simulink model "MIL4L3_SW6_V1_20220211"  (R2018b)
settings: Solver=FixedStepAuto  StartTime=0.0  StopTime=inf  FixedStep=0.001  RelTol=1e-3
PreLoadFcn:
  | A0_MILtest;
undefined symbols (not defined in the file or in its folder): Clb_ICADirect_LaneDisp_StateFive, Clb_ICADirect_LaneDisp_StateFour, Clb_ICADirect_LaneDisp_StateOne, Clb_ICADirect_LaneDisp_StateThree, Clb_ICADirect_LaneDisp_StateTwo, Clb_ICADirect_LaneDisp_StateZero, Clb_ICADirect_LaneDispSW, Clb_ICADirect_TrnLghtsCom_Switch, Clb_ICADirect_TrnLghtsCom_Value, Clb_ICADirect_TrnLghtsCrtl_Inhb, IMAP_Clb_ACU_Driver_Belt, IMAP_Clb_ACU_Driver_Belt_Over, IMAP_Clb_ACU_Passenger_Belt, IMAP_Clb_ACU_Passenger_Belt_Over, IMAP_Clb_ACU_RearLeft_Belt, IMAP_Clb_ACU_RearLeft_Belt_Over, IMAP_Clb_ACU_RearMiddle_Belt, IMAP_Clb_ACU_RearMiddle_Belt_Over, IMAP_Clb_ACU_RearRight_Belt, IMAP_Clb_ACU_RearRight_Belt_Over, IMAP_Clb_AEB_Switch, IMAP_Clb_AEB_Switch_Over, IMAP_Clb_ALC_TLC_Mode, IMAP_Clb_ALC_TLC_Mode_Over, IMAP_Clb_BCM_Battery_Voltage, IMAP_Clb_BCM_Battery_Voltage_Over, IMAP_Clb_BCM_BrakeLamp_State, IMAP_Clb_BCM_BrakeLamp_State_Over, IMAP_Clb_BCM_CHMSL_Status, IMAP_Clb_BCM_CHMSL_Status_Over, IMAP_Clb_BCM_Door_Lock_State, IMAP_Clb_BCM_Door_Lock_State_Over, IMAP_Clb_BCM_FrontWiper_State, IMAP_Clb_BCM_FrontWiper_State_Over, IMAP_Clb_BCM_FrontWiper_Switch, IMAP_Clb_BCM_FrontWiper_Switch_Over, IMAP_Clb_BCM_HazardLamp, IMAP_Clb_BCM_HazardLamp_Over, IMAP_Clb_BCM_HazardLamp_Switch, IMAP_Clb_BCM_HazardLamp_Switch_Over, IMAP_Clb_BCM_HighBeam_State, IMAP_Clb_BCM_HighBeam_State_Over, IMAP_Clb_BCM_Ignition_State, IMAP_Clb_BCM_Ignition_State_Over, IMAP_Clb_BCM_IHBC_Enabled, IMAP_Clb_BCM_IHBC_Enabled_Over, IMAP_Clb_BCM_Left_Light, IMAP_Clb_BCM_Left_Light_Over, IMAP_Clb_BCM_LeftTurn_Switch, IMAP_Clb_BCM_LeftTurn_Switch_Over, IMAP_Clb_BCM_LF_Door_State, IMAP_Clb_BCM_LF_Door_State_Over, IMAP_Clb_BCM_LowBeam_State, IMAP_Clb_BCM_LowBeam_State_Over, IMAP_Clb_BCM_LR_Door_State, IMAP_Clb_BCM_LR_Door_State_Over, IMAP_Clb_BCM_RF_Door_State, IMAP_Clb_BCM_RF_Door_State_Over, IMAP_Clb_BCM_Right_Light, IMAP_Clb_BCM_Right_Light_Over ... (+547)
libraries: CarMaker4SL x2153, simulink x292, dspstat3 x3, canmsglib x2, simulink_extras x1
(part 17 of 52)

== system MIL4L3_SW6_V1_20220211/CarMaker/VehicleControl/SDFADataLog/Subsystem53 ==
  BusCreator : BusCreator  Inputs=10
  Data Type Conversion{1..3,92} (4 alike) : DataTypeConversion  OutDataTypeStr=single
  Ground{,1..5} (6 alike) : Ground
  Read CM Dict1 : CarMaker4SL/Read CM Dict  xname=User.IO.Out.Width_S2_002  xsync=off
  Read CM Dict2 : CarMaker4SL/Read CM Dict  xname=User.IO.Out.Width_S2_003  xsync=off
  Read CM Dict3 : CarMaker4SL/Read CM Dict  xname=User.IO.Out.Width_S2_004  xsync=off
  Read CM Dict5 : CarMaker4SL/Read CM Dict  xname=User.IO.Out.Width_S2_001  xsync=off
  LFtar_Width : Outport
  wires:
  Data Type Conversion92/1 -> BusCreator/1
  Data Type Conversion3/1 -> BusCreator/4
  Data Type Conversion2/1 -> BusCreator/3
  Data Type Conversion1/1 -> BusCreator/2
  BusCreator/1 -> LFtar_Width/1
  Read CM Dict3/1 -> Data Type Conversion3/1
  Read CM Dict2/1 -> Data Type Conversion2/1
  Read CM Dict1/1 -> Data Type Conversion1/1
  Read CM Dict5/1 -> Data Type Conversion92/1
  Ground/1 -> BusCreator/5
  Ground1/1 -> BusCreator/6
  Ground2/1 -> BusCreator/7
  Ground3/1 -> BusCreator/8
  Ground4/1 -> BusCreator/9
  Ground5/1 -> BusCreator/10

== system MIL4L3_SW6_V1_20220211/CarMaker/VehicleControl/SDFADataLog/Subsystem54 ==
  BusCreator : BusCreator  Inputs=10
  Data Type Conversion{1..3,92} (4 alike) : DataTypeConversion  OutDataTypeStr=single
  Ground{,1..5} (6 alike) : Ground
  Read CM Dict1 : CarMaker4SL/Read CM Dict  xname=User.IO.Out.Length_S2_002  xsync=off
  Read CM Dict2 : CarMaker4SL/Read CM Dict  xname=User.IO.Out.Length_S2_003  xsync=off
  Read CM Dict3 : CarMaker4SL/Read CM Dict  xname=User.IO.Out.Length_S2_004  xsync=off
  Read CM Dict5 : CarMaker4SL/Read CM Dict  xname=User.IO.Out.Length_S2_001  xsync=off
  LFtar_Length : Outport
  wires:
  Data Type Conversion2/1 -> BusCreator/3
  Data Type Conversion92/1 -> BusCreator/1
  Data Type Conversion3/1 -> BusCreator/4
  Data Type Conversion1/1 -> BusCreator/2
  Ground5/1 -> BusCreator/10
  Ground4/1 -> BusCreator/9
  Ground3/1 -> BusCreator/8
  Ground2/1 -> BusCreator/7
  Ground1/1 -> BusCreator/6
  Ground/1 -> BusCreator/5
  Read CM Dict5/1 -> Data Type Conversion92/1
  Read CM Dict1/1 -> Data Type Conversion1/1
  Read CM Dict2/1 -> Data Type Conversion2/1
  Read CM Dict3/1 -> Data Type Conversion3/1
  BusCreator/1 -> LFtar_Length/1

== system MIL4L3_SW6_V1_20220211/CarMaker/VehicleControl/SDFADataLog/Subsystem55 ==
  BusCreator : BusCreator  Inputs=10
  Data Type Conversion{1..3,92} (4 alike) : DataTypeConversion  OutDataTypeStr=single
  Ground{,1..5} (6 alike) : Ground
  Read CM Dict1 : CarMaker4SL/Read CM Dict  xname=User.IO.Out.Orientation_S2_002  xsync=off
  Read CM Dict2 : CarMaker4SL/Read CM Dict  xname=User.IO.Out.Orientation_S2_003  xsync=off
  Read CM Dict3 : CarMaker4SL/Read CM Dict  xname=User.IO.Out.Orientation_S2_004  xsync=off
  Read CM Dict5 : CarMaker4SL/Read CM Dict  xname=User.IO.Out.Orientation_S2_001  xsync=off
  LFtar_Orientation : Outport
  wires:
  Data Type Conversion3/1 -> BusCreator/4
  Data Type Conversion92/1 -> BusCreator/1
  Data Type Conversion2/1 -> BusCreator/3
  Data Type Conversion1/1 -> BusCreator/2
  BusCreator/1 -> LFtar_Orientation/1
  Read CM Dict3/1 -> Data Type Conversion3/1
  Read CM Dict2/1 -> Data Type Conversion2/1
  Read CM Dict1/1 -> Data Type Conversion1/1
  Read CM Dict5/1 -> Data Type Conversion92/1
  Ground/1 -> BusCreator/5
  Ground1/1 -> BusCreator/6
  Ground2/1 -> BusCreator/7
  Ground3/1 -> BusCreator/8
  Ground4/1 -> BusCreator/9
  Ground5/1 -> BusCreator/10

== system MIL4L3_SW6_V1_20220211/CarMaker/VehicleControl/SDFADataLog/Subsystem56 ==
  BusCreator : BusCreator  Inputs=10
  Data Type Conversion{1..3,92} (4 alike) : DataTypeConversion  OutDataTypeStr=single
  Ground{,1..5} (6 alike) : Ground
  Read CM Dict1 : CarMaker4SL/Read CM Dict  xname=User.IO.Out.ExistenceProbability_S2_002  xsync=off
  Read CM Dict2 : CarMaker4SL/Read CM Dict  xname=User.IO.Out.ExistenceProbability_S2_003  xsync=off
  Read CM Dict3 : CarMaker4SL/Read CM Dict  xname=User.IO.Out.ExistenceProbability_S2_004  xsync=off
  Read CM Dict5 : CarMaker4SL/Read CM Dict  xname=User.IO.Out.ExistenceProbability_S2_001  xsync=off
  LFtar_ExistenceProbability : Outport
  wires:
  Data Type Conversion2/1 -> BusCreator/3
  Data Type Conversion92/1 -> BusCreator/1
  Data Type Conversion3/1 -> BusCreator/4
  Data Type Conversion1/1 -> BusCreator/2
  Ground5/1 -> BusCreator/10
  Ground4/1 -> BusCreator/9
  Ground3/1 -> BusCreator/8
  Ground2/1 -> BusCreator/7
  Ground1/1 -> BusCreator/6
  Ground/1 -> BusCreator/5
  Read CM Dict5/1 -> Data Type Conversion92/1
  Read CM Dict1/1 -> Data Type Conversion1/1
  Read CM Dict2/1 -> Data Type Conversion2/1
  Read CM Dict3/1 -> Data Type Conversion3/1
  BusCreator/1 -> LFtar_ExistenceProbability/1

== system MIL4L3_SW6_V1_20220211/CarMaker/VehicleControl/SDFADataLog/Subsystem57 ==
  BusCreator : BusCreator  Inputs=10
  Data Type Conversion{1..3,92} (4 alike) : DataTypeConversion  OutDataTypeStr=uint8
  Ground{,1..5} (6 alike) : Ground
  Read CM Dict1 : CarMaker4SL/Read CM Dict  xname=User.IO.Out.ClassHighest_S2_002  xsync=off
  Read CM Dict2 : CarMaker4SL/Read CM Dict  xname=User.IO.Out.ClassHighest_S2_003  xsync=off
  Read CM Dict3 : CarMaker4SL/Read CM Dict  xname=User.IO.Out.ClassHighest_S2_004  xsync=off
  Read CM Dict5 : CarMaker4SL/Read CM Dict  xname=User.IO.Out.ClassHighest_S2_001  xsync=off
  LFtar_Class : Outport
  wires:
  Data Type Conversion92/1 -> BusCreator/1
  Data Type Conversion3/1 -> BusCreator/4
  Data Type Conversion1/1 -> BusCreator/2
  Data Type Conversion2/1 -> BusCreator/3
  BusCreator/1 -> LFtar_Class/1
  Read CM Dict3/1 -> Data Type Conversion3/1
  Read CM Dict2/1 -> Data Type Conversion2/1
  Read CM Dict1/1 -> Data Type Conversion1/1
  Read CM Dict5/1 -> Data Type Conversion92/1
  Ground/1 -> BusCreator/5
  Ground1/1 -> BusCreator/6
  Ground2/1 -> BusCreator/7
  Ground3/1 -> BusCreator/8
  Ground4/1 -> BusCreator/9
  Ground5/1 -> BusCreator/10

== system MIL4L3_SW6_V1_20220211/CarMaker/VehicleControl/SDFADataLog/Subsystem58 ==
  BusCreator : BusCreator  Inputs=10
  Data Type Conversion{1..3,92} (4 alike) : DataTypeConversion  OutDataTypeStr=single
  Ground{,1..5} (6 alike) : Ground
  Read CM Dict1 : CarMaker4SL/Read CM Dict  xname=User.IO.Out.ReferencePoint_S2_002  xsync=off
  Read CM Dict2 : CarMaker4SL/Read CM Dict  xname=User.IO.Out.ReferencePoint_S2_003  xsync=off
  Read CM Dict3 : CarMaker4SL/Read CM Dict  xname=User.IO.Out.ReferencePoint_S2_004  xsync=off
  Read CM Dict5 : CarMaker4SL/Read CM Dict  xname=User.IO.Out.ReferencePoint_S2_001  xsync=off
  LFtar_ReferencePoint : Outport
  wires:
  Data Type Conversion92/1 -> BusCreator/1
  Data Type Conversion3/1 -> BusCreator/4
  Data Type Conversion2/1 -> BusCreator/3
  Data Type Conversion1/1 -> BusCreator/2
  Ground5/1 -> BusCreator/10
  Ground4/1 -> BusCreator/9
  Ground3/1 -> BusCreator/8
  Ground2/1 -> BusCreator/7
  Ground1/1 -> BusCreator/6
  Ground/1 -> BusCreator/5
  Read CM Dict5/1 -> Data Type Conversion92/1
  Read CM Dict1/1 -> Data Type Conversion1/1
  Read CM Dict2/1 -> Data Type Conversion2/1
  Read CM Dict3/1 -> Data Type Conversion3/1
  BusCreator/1 -> LFtar_ReferencePoint/1

== system MIL4L3_SW6_V1_20220211/CarMaker/VehicleControl/SDFADataLog/Subsystem59 ==
  BusCreator : BusCreator  Inputs=10
  Data Type Conversion{1..3,92} (4 alike) : DataTypeConversion  OutDataTypeStr=single
  Ground{,1..5} (6 alike) : Ground
  Read CM Dict1 : CarMaker4SL/Read CM Dict  xname=User.IO.Out.MovingState_S2_002  xsync=off
  Read CM Dict2 : CarMaker4SL/Read CM Dict  xname=User.IO.Out.MovingState_S2_003  xsync=off
  Read CM Dict3 : CarMaker4SL/Read CM Dict  xname=User.IO.Out.MovingState_S2_004  xsync=off
  Read CM Dict5 : CarMaker4SL/Read CM Dict  xname=User.IO.Out.MovingState_S2_001  xsync=off
  LFtar_MovingState : Outport
  wires:
  Data Type Conversion92/1 -> BusCreator/1
  Data Type Conversion3/1 -> BusCreator/4
  Data Type Conversion2/1 -> BusCreator/3
  Data Type Conversion1/1 -> BusCreator/2
  BusCreator/1 -> LFtar_MovingState/1
  Read CM Dict3/1 -> Data Type Conversion3/1
  Read CM Dict2/1 -> Data Type Conversion2/1
  Read CM Dict1/1 -> Data Type Conversion1/1
  Read CM Dict5/1 -> Data Type Conversion92/1
  Ground/1 -> BusCreator/5
  Ground1/1 -> BusCreator/6
  Ground2/1 -> BusCreator/7
  Ground3/1 -> BusCreator/8
  Ground4/1 -> BusCreator/9
  Ground5/1 -> BusCreator/10

== system MIL4L3_SW6_V1_20220211/CarMaker/VehicleControl/SDFADataLog/Subsystem6 ==
  Bus Creator : BusCreator  Inputs=20
  Ground{,1..15} (16 alike) : Ground
  Read CM Dict1 : CarMaker4SL/Read CM Dict  xname=User.IO.Out.IFC_obj02_HeadOrientation  xsync=off
  Read CM Dict2 : CarMaker4SL/Read CM Dict  xname=User.IO.Out.IFC_obj03_HeadOrientation  xsync=off
  Read CM Dict3 : CarMaker4SL/Read CM Dict  xname=User.IO.Out.IFC_obj04_HeadOrientation  xsync=off
  Read CM Dict4 : CarMaker4SL/Read CM Dict  xname=User.IO.Out.IFC_obj01_HeadOrientation  xsync=off
  obj_HeadOrientation : Outport
  wires:
  Bus Creator/1 -> obj_HeadOrientation/1
  Ground15/1 -> Bus Creator/20
  Ground11/1 -> Bus Creator/16
  Ground14/1 -> Bus Creator/19
  Ground12/1 -> Bus Creator/17
  Ground3/1 -> Bus Creator/8
  Ground1/1 -> Bus Creator/6
  Read CM Dict1/1 -> Bus Creator/2
  Read CM Dict4/1 -> Bus Creator/1
  Ground6/1 -> Bus Creator/11
  Ground10/1 -> Bus Creator/15
  Ground13/1 -> Bus Creator/18
  Ground2/1 -> Bus Creator/7
  Ground/1 -> Bus Creator/5
  Ground7/1 -> Bus Creator/12
  Read CM Dict3/1 -> Bus Creator/4
  Ground4/1 -> Bus Creator/9
  Ground9/1 -> Bus Creator/14
  Ground5/1 -> Bus Creator/10
  Ground8/1 -> Bus Creator/13
  Read CM Dict2/1 -> Bus Creator/3

== system MIL4L3_SW6_V1_20220211/CarMaker/VehicleControl/SDFADataLog/Subsystem61 ==
  BusCreator : BusCreator  Inputs=10
  Data Type Conversion{1..3,92} (4 alike) : DataTypeConversion  OutDataTypeStr=single
  Ground{,1..5} (6 alike) : Ground
  Read CM Dict1 : CarMaker4SL/Read CM Dict  xname=User.IO.Out.ClassHighestProb_S2_002  xsync=off
  Read CM Dict2 : CarMaker4SL/Read CM Dict  xname=User.IO.Out.ClassHighestProb_S2_003  xsync=off
  Read CM Dict3 : CarMaker4SL/Read CM Dict  xname=User.IO.Out.ClassHighestProb_S2_004  xsync=off
  Read CM Dict5 : CarMaker4SL/Read CM Dict  xname=User.IO.Out.ClassHighestProb_S2_001  xsync=off
  LFtar_ClassHighestProb : Outport
  wires:
  Data Type Conversion3/1 -> BusCreator/4
  Data Type Conversion92/1 -> BusCreator/1
  Data Type Conversion2/1 -> BusCreator/3
  Data Type Conversion1/1 -> BusCreator/2
  BusCreator/1 -> LFtar_ClassHighestProb/1
  Read CM Dict3/1 -> Data Type Conversion3/1
  Read CM Dict2/1 -> Data Type Conversion2/1
  Read CM Dict1/1 -> Data Type Conversion1/1
  Read CM Dict5/1 -> Data Type Conversion92/1
  Ground/1 -> BusCreator/5
  Ground1/1 -> BusCreator/6
  Ground2/1 -> BusCreator/7
  Ground3/1 -> BusCreator/8
  Ground4/1 -> BusCreator/9
  Ground5/1 -> BusCreator/10

== system MIL4L3_SW6_V1_20220211/CarMaker/VehicleControl/SDFADataLog/Subsystem66 ==
  BusCreator : BusCreator  Inputs=10
  Data Type Conversion{1..3,92} (4 alike) : DataTypeConversion  OutDataTypeStr=uint16
  Ground{,1..5} (6 alike) : Ground
  Read CM Dict1 : CarMaker4SL/Read CM Dict  xname=User.IO.Out.Id_S3_002  xsync=off
  Read CM Dict2 : CarMaker4SL/Read CM Dict  xname=User.IO.Out.Id_S3_003  xsync=off
  Read CM Dict3 : CarMaker4SL/Read CM Dict  xname=User.IO.Out.Id_S3_004  xsync=off
  Read CM Dict5 : CarMaker4SL/Read CM Dict  xname=User.IO.Out.Id_S3_001  xsync=off
  RFtar_id : Outport
  wires:
  Data Type Conversion92/1 -> BusCreator/1
  Data Type Conversion3/1 -> BusCreator/4
  Data Type Conversion2/1 -> BusCreator/3
  Data Type Conversion1/1 -> BusCreator/2
  BusCreator/1 -> RFtar_id/1
  Read CM Dict3/1 -> Data Type Conversion3/1
  Read CM Dict2/1 -> Data Type Conversion2/1
  Read CM Dict1/1 -> Data Type Conversion1/1
  Read CM Dict5/1 -> Data Type Conversion92/1
  Ground/1 -> BusCreator/5
  Ground1/1 -> BusCreator/6
  Ground2/1 -> BusCreator/7
  Ground3/1 -> BusCreator/8
  Ground4/1 -> BusCreator/9
  Ground5/1 -> BusCreator/10

== system MIL4L3_SW6_V1_20220211/CarMaker/VehicleControl/SDFADataLog/Subsystem67 ==
  BusCreator : BusCreator  Inputs=10
  Data Type Conversion{1..3,92} (4 alike) : DataTypeConversion  OutDataTypeStr=single
  Ground{,1..5} (6 alike) : Ground
  Read CM Dict1 : CarMaker4SL/Read CM Dict  xname=User.IO.Out.XPos_S3_002  xsync=off
  Read CM Dict2 : CarMaker4SL/Read CM Dict  xname=User.IO.Out.XPos_S3_003  xsync=off
  Read CM Dict3 : CarMaker4SL/Read CM Dict  xname=User.IO.Out.XPos_S3_004  xsync=off
  Read CM Dict5 : CarMaker4SL/Read CM Dict  xname=User.IO.Out.XPos_S3_001  xsync=off
  RFtar_Xpos : Outport
  wires:
  Data Type Conversion3/1 -> BusCreator/4
  Data Type Conversion92/1 -> BusCreator/1
  Data Type Conversion2/1 -> BusCreator/3
  Data Type Conversion1/1 -> BusCreator/2
  Ground5/1 -> BusCreator/10
  Ground4/1 -> BusCreator/9
  Ground3/1 -> BusCreator/8
  Ground2/1 -> BusCreator/7
  Ground1/1 -> BusCreator/6
  Ground/1 -> BusCreator/5
  Read CM Dict5/1 -> Data Type Conversion92/1
  Read CM Dict1/1 -> Data Type Conversion1/1
  Read CM Dict2/1 -> Data Type Conversion2/1
  Read CM Dict3/1 -> Data Type Conversion3/1
  BusCreator/1 -> RFtar_Xpos/1

== system MIL4L3_SW6_V1_20220211/CarMaker/VehicleControl/SDFADataLog/Subsystem68 ==
  BusCreator : BusCreator  Inputs=10
  Data Type Conversion{1..3,92} (4 alike) : DataTypeConversion  OutDataTypeStr=single
  Ground{,1..5} (6 alike) : Ground
  Read CM Dict1 : CarMaker4SL/Read CM Dict  xname=User.IO.Out.YPos_S3_002  xsync=off
  Read CM Dict2 : CarMaker4SL/Read CM Dict  xname=User.IO.Out.YPos_S3_003  xsync=off
  Read CM Dict3 : CarMaker4SL/Read CM Dict  xname=User.IO.Out.YPos_S3_004  xsync=off
  Read CM Dict5 : CarMaker4SL/Read CM Dict  xname=User.IO.Out.YPos_S3_001  xsync=off
  RFtar_Ypos : Outport
  wires:
  Data Type Conversion92/1 -> BusCreator/1
  Data Type Conversion2/1 -> BusCreator/3
  Data Type Conversion3/1 -> BusCreator/4
  Data Type Conversion1/1 -> BusCreator/2
  BusCreator/1 -> RFtar_Ypos/1
  Read CM Dict3/1 -> Data Type Conversion3/1
  Read CM Dict2/1 -> Data Type Conversion2/1
  Read CM Dict1/1 -> Data Type Conversion1/1
  Read CM Dict5/1 -> Data Type Conversion92/1
  Ground/1 -> BusCreator/5
  Ground1/1 -> BusCreator/6
  Ground2/1 -> BusCreator/7
  Ground3/1 -> BusCreator/8
  Ground4/1 -> BusCreator/9
  Ground5/1 -> BusCreator/10

== system MIL4L3_SW6_V1_20220211/CarMaker/VehicleControl/SDFADataLog/Subsystem69 ==
  BusCreator : BusCreator  Inputs=10
  Data Type Conversion{1..3,92} (4 alike) : DataTypeConversion  OutDataTypeStr=single
  Ground{,1..5} (6 alike) : Ground
  Read CM Dict1 : CarMaker4SL/Read CM Dict  xname=User.IO.Out.XVelocity_S3_002  xsync=off
  Read CM Dict2 : CarMaker4SL/Read CM Dict  xname=User.IO.Out.XVelocity_S3_003  xsync=off
  Read CM Dict3 : CarMaker4SL/Read CM Dict  xname=User.IO.Out.XVelocity_S3_004  xsync=off
  Read CM Dict5 : CarMaker4SL/Read CM Dict  xname=User.IO.Out.XVelocity_S3_001  xsync=off
  RFtar_Xvelocity : Outport
  wires:
  Data Type Conversion2/1 -> BusCreator/3
  Data Type Conversion1/1 -> BusCreator/2
  Data Type Conversion92/1 -> BusCreator/1
  Data Type Conversion3/1 -> BusCreator/4
  Ground5/1 -> BusCreator/10
  Ground4/1 -> BusCreator/9
  Ground3/1 -> BusCreator/8
  Ground2/1 -> BusCreator/7
  Ground1/1 -> BusCreator/6
  Ground/1 -> BusCreator/5
  Read CM Dict5/1 -> Data Type Conversion92/1
  Read CM Dict1/1 -> Data Type Conversion1/1
  Read CM Dict2/1 -> Data Type Conversion2/1
  Read CM Dict3/1 -> Data Type Conversion3/1
  BusCreator/1 -> RFtar_Xvelocity/1

== system MIL4L3_SW6_V1_20220211/CarMaker/VehicleControl/SDFADataLog/Subsystem7 ==
  Bus Creator : BusCreator  Inputs=20
  Ground{,1..15} (16 alike) : Ground
  Read CM Dict : CarMaker4SL/Read CM Dict  xname=User.IO.Out.IFC_obj01_DirIndicator  xsync=off
  Read CM Dict1 : CarMaker4SL/Read CM Dict  xname=User.IO.Out.IFC_obj02_DirIndicator  xsync=off
  Read CM Dict2 : CarMaker4SL/Read CM Dict  xname=User.IO.Out.IFC_obj03_DirIndicator  xsync=off
  Read CM Dict3 : CarMaker4SL/Read CM Dict  xname=User.IO.Out.IFC_obj04_DirIndicator  xsync=off
  obj_DirIndicator : Outport
  wires:
  Read CM Dict2/1 -> Bus Creator/3
  Ground8/1 -> Bus Creator/13
  Ground5/1 -> Bus Creator/10
  Ground9/1 -> Bus Creator/14
  Ground4/1 -> Bus Creator/9
  Read CM Dict3/1 -> Bus Creator/4
  Ground7/1 -> Bus Creator/12
  Ground/1 -> Bus Creator/5
  Ground2/1 -> Bus Creator/7
  Ground13/1 -> Bus Creator/18
  Ground10/1 -> Bus Creator/15
  Ground6/1 -> Bus Creator/11
  Read CM Dict/1 -> Bus Creator/1
  Read CM Dict1/1 -> Bus Creator/2
  Ground1/1 -> Bus Creator/6
  Ground3/1 -> Bus Creator/8
  Ground12/1 -> Bus Creator/17
  Ground14/1 -> Bus Creator/19
  Ground11/1 -> Bus Creator/16
  Ground15/1 -> Bus Creator/20
  Bus Creator/1 -> obj_DirIndicator/1

== system MIL4L3_SW6_V1_20220211/CarMaker/VehicleControl/SDFADataLog/Subsystem70 ==
  BusCreator : BusCreator  Inputs=10
  Data Type Conversion{1..3,92} (4 alike) : DataTypeConversion  OutDataTypeStr=single
  Ground{,1..5} (6 alike) : Ground
  Read CM Dict1 : CarMaker4SL/Read CM Dict  xname=User.IO.Out.YVelocity_S3_002  xsync=off
  Read CM Dict2 : CarMaker4SL/Read CM Dict  xname=User.IO.Out.YVelocity_S3_003  xsync=off
  Read CM Dict3 : CarMaker4SL/Read CM Dict  xname=User.IO.Out.YVelocity_S3_004  xsync=off
  Read CM Dict5 : CarMaker4SL/Read CM Dict  xname=User.IO.Out.YVelocity_S3_001  xsync=off
  RFtar_Yvelocity : Outport
  wires:
  Data Type Conversion92/1 -> BusCreator/1
  Data Type Conversion2/1 -> BusCreator/3
  Data Type Conversion3/1 -> BusCreator/4
  Data Type Conversion1/1 -> BusCreator/2
  BusCreator/1 -> RFtar_Yvelocity/1
  Read CM Dict3/1 -> Data Type Conversion3/1
  Read CM Dict2/1 -> Data Type Conversion2/1
  Read CM Dict1/1 -> Data Type Conversion1/1
  Read CM Dict5/1 -> Data Type Conversion92/1
  Ground/1 -> BusCreator/5
  Ground1/1 -> BusCreator/6
  Ground2/1 -> BusCreator/7
  Ground3/1 -> BusCreator/8
  Ground4/1 -> BusCreator/9
  Ground5/1 -> BusCreator/10

== system MIL4L3_SW6_V1_20220211/CarMaker/VehicleControl/SDFADataLog/Subsystem71 ==
  BusCreator : BusCreator  Inputs=10
  Data Type Conversion{1..3,92} (4 alike) : DataTypeConversion  OutDataTypeStr=single
  Ground{,1..5} (6 alike) : Ground
  Read CM Dict1 : CarMaker4SL/Read CM Dict  xname=User.IO.Out.XAcceleration_S3_002  xsync=off
  Read CM Dict2 : CarMaker4SL/Read CM Dict  xname=User.IO.Out.XAcceleration_S3_003  xsync=off
  Read CM Dict3 : CarMaker4SL/Read CM Dict  xname=User.IO.Out.XAcceleration_S3_004  xsync=off
  Read CM Dict5 : CarMaker4SL/Read CM Dict  xname=User.IO.Out.XAcceleration_S3_001  xsync=off
  RFtar_Xacceleration : Outport
  wires:
  Data Type Conversion92/1 -> BusCreator/1
  Data Type Conversion3/1 -> BusCreator/4
  Data Type Conversion1/1 -> BusCreator/2
  Data Type Conversion2/1 -> BusCreator/3
  Ground5/1 -> BusCreator/10
  Ground4/1 -> BusCreator/9
  Ground3/1 -> BusCreator/8
  Ground2/1 -> BusCreator/7
  Ground1/1 -> BusCreator/6
  Ground/1 -> BusCreator/5
  Read CM Dict5/1 -> Data Type Conversion92/1
  Read CM Dict1/1 -> Data Type Conversion1/1
  Read CM Dict2/1 -> Data Type Conversion2/1
  Read CM Dict3/1 -> Data Type Conversion3/1
  BusCreator/1 -> RFtar_Xacceleration/1

== system MIL4L3_SW6_V1_20220211/CarMaker/VehicleControl/SDFADataLog/Subsystem72 ==
  BusCreator : BusCreator  Inputs=10
  Data Type Conversion{1..3,92} (4 alike) : DataTypeConversion  OutDataTypeStr=single
  Ground{,1..5} (6 alike) : Ground
  Read CM Dict1 : CarMaker4SL/Read CM Dict  xname=User.IO.Out.YAcceleration_S3_002  xsync=off
  Read CM Dict2 : CarMaker4SL/Read CM Dict  xname=User.IO.Out.YAcceleration_S3_003  xsync=off
  Read CM Dict3 : CarMaker4SL/Read CM Dict  xname=User.IO.Out.YAcceleration_S3_004  xsync=off
  Read CM Dict5 : CarMaker4SL/Read CM Dict  xname=User.IO.Out.YAcceleration_S3_001  xsync=off
  RFtar_Yacceleration : Outport
  wires:
  Data Type Conversion92/1 -> BusCreator/1
  Data Type Conversion3/1 -> BusCreator/4
  Data Type Conversion2/1 -> BusCreator/3
  Data Type Conversion1/1 -> BusCreator/2
  BusCreator/1 -> RFtar_Yacceleration/1
  Read CM Dict3/1 -> Data Type Conversion3/1
  Read CM Dict2/1 -> Data Type Conversion2/1
  Read CM Dict1/1 -> Data Type Conversion1/1
  Read CM Dict5/1 -> Data Type Conversion92/1
  Ground/1 -> BusCreator/5
  Ground1/1 -> BusCreator/6
  Ground2/1 -> BusCreator/7
  Ground3/1 -> BusCreator/8
  Ground4/1 -> BusCreator/9
  Ground5/1 -> BusCreator/10

== system MIL4L3_SW6_V1_20220211/CarMaker/VehicleControl/SDFADataLog/Subsystem73 ==
  BusCreator : BusCreator  Inputs=10
  Data Type Conversion{1..3,92} (4 alike) : DataTypeConversion  OutDataTypeStr=single
  Ground{,1..5} (6 alike) : Ground
  Read CM Dict1 : CarMaker4SL/Read CM Dict  xname=User.IO.Out.Width_S3_002  xsync=off
  Read CM Dict2 : CarMaker4SL/Read CM Dict  xname=User.IO.Out.Width_S3_003  xsync=off
  Read CM Dict3 : CarMaker4SL/Read CM Dict  xname=User.IO.Out.Width_S3_004  xsync=off
  Read CM Dict5 : CarMaker4SL/Read CM Dict  xname=User.IO.Out.Width_S3_001  xsync=off
  RFtar_Width : Outport
  wires:
  Data Type Conversion92/1 -> BusCreator/1
  Data Type Conversion2/1 -> BusCreator/3
  Data Type Conversion1/1 -> BusCreator/2
  Data Type Conversion3/1 -> BusCreator/4
  Ground5/1 -> BusCreator/10
  Ground4/1 -> BusCreator/9
  Ground3/1 -> BusCreator/8
  Ground2/1 -> BusCreator/7
  Ground1/1 -> BusCreator/6
  Ground/1 -> BusCreator/5
  Read CM Dict5/1 -> Data Type Conversion92/1
  Read CM Dict1/1 -> Data Type Conversion1/1
  Read CM Dict2/1 -> Data Type Conversion2/1
  Read CM Dict3/1 -> Data Type Conversion3/1
  BusCreator/1 -> RFtar_Width/1

== system MIL4L3_SW6_V1_20220211/CarMaker/VehicleControl/SDFADataLog/Subsystem74 ==
  BusCreator : BusCreator  Inputs=10
  Data Type Conversion{1..3,92} (4 alike) : DataTypeConversion  OutDataTypeStr=single
  Ground{,1..5} (6 alike) : Ground
  Read CM Dict1 : CarMaker4SL/Read CM Dict  xname=User.IO.Out.Length_S3_002  xsync=off
  Read CM Dict2 : CarMaker4SL/Read CM Dict  xname=User.IO.Out.Length_S3_003  xsync=off
  Read CM Dict3 : CarMaker4SL/Read CM Dict  xname=User.IO.Out.Length_S3_004  xsync=off
  Read CM Dict5 : CarMaker4SL/Read CM Dict  xname=User.IO.Out.Length_S3_001  xsync=off
  RFtar_Length : Outport
  wires:
  Data Type Conversion2/1 -> BusCreator/3
  Data Type Conversion3/1 -> BusCreator/4
  Data Type Conversion92/1 -> BusCreator/1
  Data Type Conversion1/1 -> BusCreator/2
  BusCreator/1 -> RFtar_Length/1
  Read CM Dict3/1 -> Data Type Conversion3/1
  Read CM Dict2/1 -> Data Type Conversion2/1
  Read CM Dict1/1 -> Data Type Conversion1/1
  Read CM Dict5/1 -> Data Type Conversion92/1
  Ground/1 -> BusCreator/5
  Ground1/1 -> BusCreator/6
  Ground2/1 -> BusCreator/7
  Ground3/1 -> BusCreator/8
  Ground4/1 -> BusCreator/9
  Ground5/1 -> BusCreator/10

== system MIL4L3_SW6_V1_20220211/CarMaker/VehicleControl/SDFADataLog/Subsystem75 ==
  BusCreator : BusCreator  Inputs=10
  Data Type Conversion{1..3,92} (4 alike) : DataTypeConversion  OutDataTypeStr=single
  Ground{,1..5} (6 alike) : Ground
  Read CM Dict1 : CarMaker4SL/Read CM Dict  xname=User.IO.Out.Orientation_S3_002  xsync=off
  Read CM Dict2 : CarMaker4SL/Read CM Dict  xname=User.IO.Out.Orientation_S3_003  xsync=off
  Read CM Dict3 : CarMaker4SL/Read CM Dict  xname=User.IO.Out.Orientation_S3_004  xsync=off
  Read CM Dict5 : CarMaker4SL/Read CM Dict  xname=User.IO.Out.Orientation_S3_001  xsync=off
  RFtar_Orientation : Outport
  wires:
  Data Type Conversion92/1 -> BusCreator/1
  Data Type Conversion2/1 -> BusCreator/3
  Data Type Conversion1/1 -> BusCreator/2
  Data Type Conversion3/1 -> BusCreator/4
  Ground5/1 -> BusCreator/10
  Ground4/1 -> BusCreator/9
  Ground3/1 -> BusCreator/8
  Ground2/1 -> BusCreator/7
  Ground1/1 -> BusCreator/6
  Ground/1 -> BusCreator/5
  Read CM Dict5/1 -> Data Type Conversion92/1
  Read CM Dict1/1 -> Data Type Conversion1/1
  Read CM Dict2/1 -> Data Type Conversion2/1
  Read CM Dict3/1 -> Data Type Conversion3/1
  BusCreator/1 -> RFtar_Orientation/1

== system MIL4L3_SW6_V1_20220211/CarMaker/VehicleControl/SDFADataLog/Subsystem76 ==
  BusCreator : BusCreator  Inputs=10
  Data Type Conversion{1..3,92} (4 alike) : DataTypeConversion  OutDataTypeStr=single
  Ground{,1..5} (6 alike) : Ground
  Read CM Dict1 : CarMaker4SL/Read CM Dict  xname=User.IO.Out.ExistenceProbability_S3_002  xsync=off
  Read CM Dict2 : CarMaker4SL/Read CM Dict  xname=User.IO.Out.ExistenceProbability_S3_003  xsync=off
  Read CM Dict3 : CarMaker4SL/Read CM Dict  xname=User.IO.Out.ExistenceProbability_S3_004  xsync=off
  Read CM Dict5 : CarMaker4SL/Read CM Dict  xname=User.IO.Out.ExistenceProbability_S3_001  xsync=off
  RFtar_ExistenceProbability : Outport
  wires:
  Data Type Conversion2/1 -> BusCreator/3
  Data Type Conversion3/1 -> BusCreator/4
  Data Type Conversion1/1 -> BusCreator/2
  Data Type Conversion92/1 -> BusCreator/1
  BusCreator/1 -> RFtar_ExistenceProbability/1
  Read CM Dict3/1 -> Data Type Conversion3/1
  Read CM Dict2/1 -> Data Type Conversion2/1
  Read CM Dict1/1 -> Data Type Conversion1/1
  Read CM Dict5/1 -> Data Type Conversion92/1
  Ground/1 -> BusCreator/5
  Ground1/1 -> BusCreator/6
  Ground2/1 -> BusCreator/7
  Ground3/1 -> BusCreator/8
  Ground4/1 -> BusCreator/9
  Ground5/1 -> BusCreator/10

== system MIL4L3_SW6_V1_20220211/CarMaker/VehicleControl/SDFADataLog/Subsystem77 ==
  BusCreator : BusCreator  Inputs=10
  Data Type Conversion{1..3,92} (4 alike) : DataTypeConversion  OutDataTypeStr=uint8
  Ground{,1..5} (6 alike) : Ground
  Read CM Dict1 : CarMaker4SL/Read CM Dict  xname=User.IO.Out.ClassHighest_S3_002  xsync=off
  Read CM Dict2 : CarMaker4SL/Read CM Dict  xname=User.IO.Out.ClassHighest_S3_003  xsync=off
  Read CM Dict3 : CarMaker4SL/Read CM Dict  xname=User.IO.Out.ClassHighest_S3_004  xsync=off
  Read CM Dict5 : CarMaker4SL/Read CM Dict  xname=User.IO.Out.ClassHighest_S3_001  xsync=off
  RFtar_Class : Outport
  wires:
  Data Type Conversion3/1 -> BusCreator/4
  Data Type Conversion2/1 -> BusCreator/3
  Data Type Conversion92/1 -> BusCreator/1
  Data Type Conversion1/1 -> BusCreator/2
  Ground5/1 -> BusCreator/10
  Ground4/1 -> BusCreator/9
  Ground3/1 -> BusCreator/8
  Ground2/1 -> BusCreator/7
  Ground1/1 -> BusCreator/6
  Ground/1 -> BusCreator/5
  Read CM Dict5/1 -> Data Type Conversion92/1
  Read CM Dict1/1 -> Data Type Conversion1/1
  Read CM Dict2/1 -> Data Type Conversion2/1
  Read CM Dict3/1 -> Data Type Conversion3/1
  BusCreator/1 -> RFtar_Class/1

== system MIL4L3_SW6_V1_20220211/CarMaker/VehicleControl/SDFADataLog/Subsystem78 ==
  BusCreator : BusCreator  Inputs=10
  Data Type Conversion{1..3,92} (4 alike) : DataTypeConversion  OutDataTypeStr=single
  Ground{,1..5} (6 alike) : Ground
  Read CM Dict1 : CarMaker4SL/Read CM Dict  xname=User.IO.Out.ReferencePoint_S3_002  xsync=off
  Read CM Dict2 : CarMaker4SL/Read CM Dict  xname=User.IO.Out.ReferencePoint_S3_003  xsync=off
  Read CM Dict3 : CarMaker4SL/Read CM Dict  xname=User.IO.Out.ReferencePoint_S3_004  xsync=off
  Read CM Dict5 : CarMaker4SL/Read CM Dict  xname=User.IO.Out.ReferencePoint_S3_001  xsync=off
  RFtar_ReferencePoint : Outport
  wires:
  Data Type Conversion1/1 -> BusCreator/2
  Data Type Conversion3/1 -> BusCreator/4
  Data Type Conversion2/1 -> BusCreator/3
  Data Type Conversion92/1 -> BusCreator/1
  BusCreator/1 -> RFtar_ReferencePoint/1
  Read CM Dict3/1 -> Data Type Conversion3/1
  Read CM Dict2/1 -> Data Type Conversion2/1
  Read CM Dict1/1 -> Data Type Conversion1/1
  Read CM Dict5/1 -> Data Type Conversion92/1
  Ground/1 -> BusCreator/5
  Ground1/1 -> BusCreator/6
  Ground2/1 -> BusCreator/7
  Ground3/1 -> BusCreator/8
  Ground4/1 -> BusCreator/9
  Ground5/1 -> BusCreator/10

== system MIL4L3_SW6_V1_20220211/CarMaker/VehicleControl/SDFADataLog/Subsystem79 ==
  BusCreator : BusCreator  Inputs=10
  Data Type Conversion{1..3,92} (4 alike) : DataTypeConversion  OutDataTypeStr=single
  Ground{,1..5} (6 alike) : Ground
  Read CM Dict1 : CarMaker4SL/Read CM Dict  xname=User.IO.Out.MovingState_S3_002  xsync=off
  Read CM Dict2 : CarMaker4SL/Read CM Dict  xname=User.IO.Out.MovingState_S3_003  xsync=off
  Read CM Dict3 : CarMaker4SL/Read CM Dict  xname=User.IO.Out.MovingState_S3_004  xsync=off
  Read CM Dict5 : CarMaker4SL/Read CM Dict  xname=User.IO.Out.MovingState_S3_001  xsync=off
  RFtar_MovingState : Outport
  wires:
  Data Type Conversion3/1 -> BusCreator/4
  Data Type Conversion92/1 -> BusCreator/1
  Data Type Conversion2/1 -> BusCreator/3
  Data Type Conversion1/1 -> BusCreator/2
  Ground5/1 -> BusCreator/10
  Ground4/1 -> BusCreator/9
  Ground3/1 -> BusCreator/8
  Ground2/1 -> BusCreator/7
  Ground1/1 -> BusCreator/6
  Ground/1 -> BusCreator/5
  Read CM Dict5/1 -> Data Type Conversion92/1
  Read CM Dict1/1 -> Data Type Conversion1/1
  Read CM Dict2/1 -> Data Type Conversion2/1
  Read CM Dict3/1 -> Data Type Conversion3/1
  BusCreator/1 -> RFtar_MovingState/1

== system MIL4L3_SW6_V1_20220211/CarMaker/VehicleControl/SDFADataLog/Subsystem8 ==
  Bus Creator : BusCreator  Inputs=20
  Ground{,1..15} (16 alike) : Ground
  Read CM Dict : CarMaker4SL/Read CM Dict  xname=User.IO.Out.IFC_obj01_angle_rate  xsync=off
  Read CM Dict1 : CarMaker4SL/Read CM Dict  xname=User.IO.Out.IFC_obj02_angle_rate  xsync=off
  Read CM Dict2 : CarMaker4SL/Read CM Dict  xname=User.IO.Out.IFC_obj03_angle_rate  xsync=off
  Read CM Dict3 : CarMaker4SL/Read CM Dict  xname=User.IO.Out.IFC_obj04_angle_rate  xsync=off
  obj_angle_rate : Outport
  wires:
  Read CM Dict2/1 -> Bus Creator/3
  Ground8/1 -> Bus Creator/13
  Ground5/1 -> Bus Creator/10
  Ground9/1 -> Bus Creator/14
  Ground4/1 -> Bus Creator/9
  Read CM Dict3/1 -> Bus Creator/4
  Ground7/1 -> Bus Creator/12
  Ground/1 -> Bus Creator/5
  Ground2/1 -> Bus Creator/7
  Ground13/1 -> Bus Creator/18
  Ground10/1 -> Bus Creator/15
  Ground6/1 -> Bus Creator/11
  Read CM Dict/1 -> Bus Creator/1
  Read CM Dict1/1 -> Bus Creator/2
  Ground1/1 -> Bus Creator/6
  Ground3/1 -> Bus Creator/8
  Ground12/1 -> Bus Creator/17
  Ground14/1 -> Bus Creator/19
  Ground11/1 -> Bus Creator/16
  Ground15/1 -> Bus Creator/20
  Bus Creator/1 -> obj_angle_rate/1

== system MIL4L3_SW6_V1_20220211/CarMaker/VehicleControl/SDFADataLog/Subsystem81 ==
  BusCreator : BusCreator  Inputs=10
  Data Type Conversion{1..3,92} (4 alike) : DataTypeConversion  OutDataTypeStr=single
  Ground{,1..5} (6 alike) : Ground
  Read CM Dict1 : CarMaker4SL/Read CM Dict  xname=User.IO.Out.ClassHighestProb_S3_002  xsync=off
  Read CM Dict2 : CarMaker4SL/Read CM Dict  xname=User.IO.Out.ClassHighestProb_S3_003  xsync=off
  Read CM Dict3 : CarMaker4SL/Read CM Dict  xname=User.IO.Out.ClassHighestProb_S3_004  xsync=off
  Read CM Dict5 : CarMaker4SL/Read CM Dict  xname=User.IO.Out.ClassHighestProb_S3_001  xsync=off
  RFtar_ClassHighestProb : Outport
  wires:
  Data Type Conversion92/1 -> BusCreator/1
  Data Type Conversion2/1 -> BusCreator/3
  Data Type Conversion3/1 -> BusCreator/4
  Data Type Conversion1/1 -> BusCreator/2
  Ground5/1 -> BusCreator/10
  Ground4/1 -> BusCreator/9
  Ground3/1 -> BusCreator/8
  Ground2/1 -> BusCreator/7
  Ground1/1 -> BusCreator/6
  Ground/1 -> BusCreator/5
  Read CM Dict5/1 -> Data Type Conversion92/1
  Read CM Dict1/1 -> Data Type Conversion1/1
  Read CM Dict2/1 -> Data Type Conversion2/1
  Read CM Dict3/1 -> Data Type Conversion3/1
  BusCreator/1 -> RFtar_ClassHighestProb/1

== system MIL4L3_SW6_V1_20220211/CarMaker/VehicleControl/SDFADataLog/Subsystem85 ==
  BusCreator : BusCreator  Inputs=10
  Data Type Conversion{1..3,92} (4 alike) : DataTypeConversion  OutDataTypeStr=uint16
  Ground{,1..5} (6 alike) : Ground
  Read CM Dict1 : CarMaker4SL/Read CM Dict  xname=User.IO.Out.Id_S0_002  xsync=off
  Read CM Dict2 : CarMaker4SL/Read CM Dict  xname=User.IO.Out.Id_S0_003  xsync=off
  Read CM Dict3 : CarMaker4SL/Read CM Dict  xname=User.IO.Out.Id_S0_004  xsync=off
  Read CM Dict5 : CarMaker4SL/Read CM Dict  xname=User.IO.Out.Id_S0_001  xsync=off
  LBtar_id : Outport
  wires:
  Data Type Conversion92/1 -> BusCreator/1
  Data Type Conversion3/1 -> BusCreator/4
  Data Type Conversion2/1 -> BusCreator/3
  Data Type Conversion1/1 -> BusCreator/2
  Ground5/1 -> BusCreator/10
  Ground4/1 -> BusCreator/9
  Ground3/1 -> BusCreator/8
  Ground2/1 -> BusCreator/7
  Ground1/1 -> BusCreator/6
  Ground/1 -> BusCreator/5
  Read CM Dict5/1 -> Data Type Conversion92/1
  Read CM Dict1/1 -> Data Type Conversion1/1
  Read CM Dict2/1 -> Data Type Conversion2/1
  Read CM Dict3/1 -> Data Type Conversion3/1
  BusCreator/1 -> LBtar_id/1

== system MIL4L3_SW6_V1_20220211/CarMaker/VehicleControl/SDFADataLog/Subsystem86 ==
  BusCreator : BusCreator  Inputs=10
  Data Type Conversion{1..3,92} (4 alike) : DataTypeConversion  OutDataTypeStr=single
  Ground{,1..5} (6 alike) : Ground
  Read CM Dict1 : CarMaker4SL/Read CM Dict  xname=User.IO.Out.XPos_S0_002  xsync=off
  Read CM Dict2 : CarMaker4SL/Read CM Dict  xname=User.IO.Out.XPos_S0_003  xsync=off
  Read CM Dict3 : CarMaker4SL/Read CM Dict  xname=User.IO.Out.XPos_S0_004  xsync=off
  Read CM Dict5 : CarMaker4SL/Read CM Dict  xname=User.IO.Out.XPos_S0_001  xsync=off
  LBtar_Xpos : Outport
  wires:
  BusCreator/1 -> LBtar_Xpos/1
  Read CM Dict3/1 -> Data Type Conversion3/1
  Read CM Dict2/1 -> Data Type Conversion2/1
  Read CM Dict1/1 -> Data Type Conversion1/1
  Read CM Dict5/1 -> Data Type Conversion92/1
  Ground/1 -> BusCreator/5
  Ground1/1 -> BusCreator/6
  Ground2/1 -> BusCreator/7
  Ground3/1 -> BusCreator/8
  Ground4/1 -> BusCreator/9
  Ground5/1 -> BusCreator/10
  Data Type Conversion92/1 -> BusCreator/1
  Data Type Conversion1/1 -> BusCreator/2
  Data Type Conversion2/1 -> BusCreator/3
  Data Type Conversion3/1 -> BusCreator/4

== system MIL4L3_SW6_V1_20220211/CarMaker/VehicleControl/SDFADataLog/Subsystem87 ==
  BusCreator : BusCreator  Inputs=10
  Data Type Conversion{1..3,92} (4 alike) : DataTypeConversion  OutDataTypeStr=single
  Ground{,1..5} (6 alike) : Ground
  Read CM Dict1 : CarMaker4SL/Read CM Dict  xname=User.IO.Out.YPos_S0_002  xsync=off
  Read CM Dict2 : CarMaker4SL/Read CM Dict  xname=User.IO.Out.YPos_S0_003  xsync=off
  Read CM Dict3 : CarMaker4SL/Read CM Dict  xname=User.IO.Out.YPos_S0_004  xsync=off
  Read CM Dict5 : CarMaker4SL/Read CM Dict  xname=User.IO.Out.YPos_S0_001  xsync=off
  LBtar_Ypos : Outport
  wires:
  Data Type Conversion2/1 -> BusCreator/3
  Data Type Conversion92/1 -> BusCreator/1
  Data Type Conversion3/1 -> BusCreator/4
  Data Type Conversion1/1 -> BusCreator/2
  Ground5/1 -> BusCreator/10
  Ground4/1 -> BusCreator/9
  Ground3/1 -> BusCreator/8
  Ground2/1 -> BusCreator/7
  Ground1/1 -> BusCreator/6
  Ground/1 -> BusCreator/5
  Read CM Dict5/1 -> Data Type Conversion92/1
  Read CM Dict1/1 -> Data Type Conversion1/1
  Read CM Dict2/1 -> Data Type Conversion2/1
  Read CM Dict3/1 -> Data Type Conversion3/1
  BusCreator/1 -> LBtar_Ypos/1

== system MIL4L3_SW6_V1_20220211/CarMaker/VehicleControl/SDFADataLog/Subsystem88 ==
  BusCreator : BusCreator  Inputs=10
  Data Type Conversion{1..3,92} (4 alike) : DataTypeConversion  OutDataTypeStr=single
  Ground{,1..5} (6 alike) : Ground
  Read CM Dict1 : CarMaker4SL/Read CM Dict  xname=User.IO.Out.XVelocity_S0_002  xsync=off
  Read CM Dict2 : CarMaker4SL/Read CM Dict  xname=User.IO.Out.XVelocity_S0_003  xsync=off
  Read CM Dict3 : CarMaker4SL/Read CM Dict  xname=User.IO.Out.XVelocity_S0_004  xsync=off
  Read CM Dict5 : CarMaker4SL/Read CM Dict  xname=User.IO.Out.XVelocity_S0_001  xsync=off
  LBtar_Xvelocity : Outport
  wires:
  Data Type Conversion92/1 -> BusCreator/1
  Data Type Conversion2/1 -> BusCreator/3
  Data Type Conversion3/1 -> BusCreator/4
  Data Type Conversion1/1 -> BusCreator/2
  BusCreator/1 -> LBtar_Xvelocity/1
  Read CM Dict3/1 -> Data Type Conversion3/1
  Read CM Dict2/1 -> Data Type Conversion2/1
  Read CM Dict1/1 -> Data Type Conversion1/1
  Read CM Dict5/1 -> Data Type Conversion92/1
  Ground/1 -> BusCreator/5
  Ground1/1 -> BusCreator/6
  Ground2/1 -> BusCreator/7
  Ground3/1 -> BusCreator/8
  Ground4/1 -> BusCreator/9
  Ground5/1 -> BusCreator/10

== system MIL4L3_SW6_V1_20220211/CarMaker/VehicleControl/SDFADataLog/Subsystem89 ==
  BusCreator : BusCreator  Inputs=10
  Data Type Conversion{1..3,92} (4 alike) : DataTypeConversion  OutDataTypeStr=single
  Ground{,1..5} (6 alike) : Ground
  Read CM Dict1 : CarMaker4SL/Read CM Dict  xname=User.IO.Out.YVelocity_S0_002  xsync=off
  Read CM Dict2 : CarMaker4SL/Read CM Dict  xname=User.IO.Out.YVelocity_S0_003  xsync=off
  Read CM Dict3 : CarMaker4SL/Read CM Dict  xname=User.IO.Out.YVelocity_S0_004  xsync=off
  Read CM Dict5 : CarMaker4SL/Read CM Dict  xname=User.IO.Out.YVelocity_S0_001  xsync=off
  LBtar_Yvelocity : Outport
  wires:
  Data Type Conversion92/1 -> BusCreator/1
  Data Type Conversion2/1 -> BusCreator/3
  Data Type Conversion3/1 -> BusCreator/4
  Data Type Conversion1/1 -> BusCreator/2
  Ground5/1 -> BusCreator/10
  Ground4/1 -> BusCreator/9
  Ground3/1 -> BusCreator/8
  Ground2/1 -> BusCreator/7
  Ground1/1 -> BusCreator/6
  Ground/1 -> BusCreator/5
  Read CM Dict5/1 -> Data Type Conversion92/1
  Read CM Dict1/1 -> Data Type Conversion1/1
  Read CM Dict2/1 -> Data Type Conversion2/1
  Read CM Dict3/1 -> Data Type Conversion3/1
  BusCreator/1 -> LBtar_Yvelocity/1

== system MIL4L3_SW6_V1_20220211/CarMaker/VehicleControl/SDFADataLog/Subsystem9 ==
  Bus Creator : BusCreator  Inputs=20
  Ground{,1..15} (16 alike) : Ground
  Read CM Dict : CarMaker4SL/Read CM Dict  xname=User.IO.Out.IFC_obj01_angle_3D  xsync=off
  Read CM Dict1 : CarMaker4SL/Read CM Dict  xname=User.IO.Out.IFC_obj02_angle_3D  xsync=off
  Read CM Dict2 : CarMaker4SL/Read CM Dict  xname=User.IO.Out.IFC_obj03_angle_3D  xsync=off
  Read CM Dict3 : CarMaker4SL/Read CM Dict  xname=User.IO.Out.IFC_obj04_angle_3D  xsync=off
  obj_angle_3D : Outport
  wires:
  Bus Creator/1 -> obj_angle_3D/1
  Ground15/1 -> Bus Creator/20
  Ground11/1 -> Bus Creator/16
  Ground14/1 -> Bus Creator/19
  Ground12/1 -> Bus Creator/17
  Ground3/1 -> Bus Creator/8
  Ground1/1 -> Bus Creator/6
  Read CM Dict1/1 -> Bus Creator/2
  Read CM Dict/1 -> Bus Creator/1
  Ground6/1 -> Bus Creator/11
  Ground10/1 -> Bus Creator/15
  Ground13/1 -> Bus Creator/18
  Ground2/1 -> Bus Creator/7
  Ground/1 -> Bus Creator/5
  Ground7/1 -> Bus Creator/12
  Read CM Dict3/1 -> Bus Creator/4
  Ground4/1 -> Bus Creator/9
  Ground9/1 -> Bus Creator/14
  Ground5/1 -> Bus Creator/10
  Ground8/1 -> Bus Creator/13
  Read CM Dict2/1 -> Bus Creator/3

== system MIL4L3_SW6_V1_20220211/CarMaker/VehicleControl/SDFADataLog/Subsystem90 ==
  BusCreator : BusCreator  Inputs=10
  Data Type Conversion{1..3,92} (4 alike) : DataTypeConversion  OutDataTypeStr=single
  Ground{,1..5} (6 alike) : Ground
  Read CM Dict1 : CarMaker4SL/Read CM Dict  xname=User.IO.Out.XAcceleration_S0_002  xsync=off
  Read CM Dict2 : CarMaker4SL/Read CM Dict  xname=User.IO.Out.XAcceleration_S0_003  xsync=off
  Read CM Dict3 : CarMaker4SL/Read CM Dict  xname=User.IO.Out.XAcceleration_S0_004  xsync=off
  Read CM Dict5 : CarMaker4SL/Read CM Dict  xname=User.IO.Out.XAcceleration_S0_001  xsync=off
  LBtar_Xacceleration : Outport
  wires:
  Data Type Conversion92/1 -> BusCreator/1
  Data Type Conversion2/1 -> BusCreator/3
  Data Type Conversion3/1 -> BusCreator/4
  Data Type Conversion1/1 -> BusCreator/2
  BusCreator/1 -> LBtar_Xacceleration/1
  Read CM Dict3/1 -> Data Type Conversion3/1
  Read CM Dict2/1 -> Data Type Conversion2/1
  Read CM Dict1/1 -> Data Type Conversion1/1
  Read CM Dict5/1 -> Data Type Conversion92/1
  Ground/1 -> BusCreator/5
  Ground1/1 -> BusCreator/6
  Ground2/1 -> BusCreator/7
  Ground3/1 -> BusCreator/8
  Ground4/1 -> BusCreator/9
  Ground5/1 -> BusCreator/10

== system MIL4L3_SW6_V1_20220211/CarMaker/VehicleControl/SDFADataLog/Subsystem91 ==
  BusCreator : BusCreator  Inputs=10
  Data Type Conversion{1..3,92} (4 alike) : DataTypeConversion  OutDataTypeStr=single
  Ground{,1..5} (6 alike) : Ground
  Read CM Dict1 : CarMaker4SL/Read CM Dict  xname=User.IO.Out.YAcceleration_S0_002  xsync=off
  Read CM Dict2 : CarMaker4SL/Read CM Dict  xname=User.IO.Out.YAcceleration_S0_003  xsync=off
  Read CM Dict3 : CarMaker4SL/Read CM Dict  xname=User.IO.Out.YAcceleration_S0_004  xsync=off
  Read CM Dict5 : CarMaker4SL/Read CM Dict  xname=User.IO.Out.YAcceleration_S0_001  xsync=off
  LBtar_Yacceleration : Outport
  wires:
  Data Type Conversion92/1 -> BusCreator/1
  Data Type Conversion3/1 -> BusCreator/4
  Data Type Conversion2/1 -> BusCreator/3
  Data Type Conversion1/1 -> BusCreator/2
  Ground5/1 -> BusCreator/10
  Ground4/1 -> BusCreator/9
  Ground3/1 -> BusCreator/8
  Ground2/1 -> BusCreator/7
  Ground1/1 -> BusCreator/6
  Ground/1 -> BusCreator/5
  Read CM Dict5/1 -> Data Type Conversion92/1
  Read CM Dict1/1 -> Data Type Conversion1/1
  Read CM Dict2/1 -> Data Type Conversion2/1
  Read CM Dict3/1 -> Data Type Conversion3/1
  BusCreator/1 -> LBtar_Yacceleration/1

== system MIL4L3_SW6_V1_20220211/CarMaker/VehicleControl/SDFADataLog/Subsystem92 ==
  BusCreator : BusCreator  Inputs=10
  Data Type Conversion{1..3,92} (4 alike) : DataTypeConversion  OutDataTypeStr=single
  Ground{,1..5} (6 alike) : Ground
  Read CM Dict1 : CarMaker4SL/Read CM Dict  xname=User.IO.Out.Width_S0_002  xsync=off
  Read CM Dict2 : CarMaker4SL/Read CM Dict  xname=User.IO.Out.Width_S0_003  xsync=off
  Read CM Dict3 : CarMaker4SL/Read CM Dict  xname=User.IO.Out.Width_S0_004  xsync=off
  Read CM Dict5 : CarMaker4SL/Read CM Dict  xname=User.IO.Out.Width_S0_001  xsync=off
  LBtar_Width : Outport
  wires:
  Data Type Conversion92/1 -> BusCreator/1
  Data Type Conversion3/1 -> BusCreator/4
  Data Type Conversion2/1 -> BusCreator/3
  Data Type Conversion1/1 -> BusCreator/2
  BusCreator/1 -> LBtar_Width/1
  Read CM Dict3/1 -> Data Type Conversion3/1
  Read CM Dict2/1 -> Data Type Conversion2/1
  Read CM Dict1/1 -> Data Type Conversion1/1
  Read CM Dict5/1 -> Data Type Conversion92/1
  Ground/1 -> BusCreator/5
  Ground1/1 -> BusCreator/6
  Ground2/1 -> BusCreator/7
  Ground3/1 -> BusCreator/8
  Ground4/1 -> BusCreator/9
  Ground5/1 -> BusCreator/10

== system MIL4L3_SW6_V1_20220211/CarMaker/VehicleControl/SDFADataLog/Subsystem93 ==
  BusCreator : BusCreator  Inputs=10
  Data Type Conversion{1..3,92} (4 alike) : DataTypeConversion  OutDataTypeStr=single
  Ground{,1..5} (6 alike) : Ground
  Read CM Dict1 : CarMaker4SL/Read CM Dict  xname=User.IO.Out.Length_S0_002  xsync=off
  Read CM Dict2 : CarMaker4SL/Read CM Dict  xname=User.IO.Out.Length_S0_003  xsync=off
  Read CM Dict3 : CarMaker4SL/Read CM Dict  xname=User.IO.Out.Length_S0_004  xsync=off
  Read CM Dict5 : CarMaker4SL/Read CM Dict  xname=User.IO.Out.Length_S0_001  xsync=off
  LBtar_Length : Outport
  wires:
  Data Type Conversion92/1 -> BusCreator/1
  Data Type Conversion2/1 -> BusCreator/3
  Data Type Conversion1/1 -> BusCreator/2
  Data Type Conversion3/1 -> BusCreator/4
  Ground5/1 -> BusCreator/10
  Ground4/1 -> BusCreator/9
  Ground3/1 -> BusCreator/8
  Ground2/1 -> BusCreator/7
  Ground1/1 -> BusCreator/6
  Ground/1 -> BusCreator/5
  Read CM Dict5/1 -> Data Type Conversion92/1
  Read CM Dict1/1 -> Data Type Conversion1/1
  Read CM Dict2/1 -> Data Type Conversion2/1
  Read CM Dict3/1 -> Data Type Conversion3/1
  BusCreator/1 -> LBtar_Length/1

== system MIL4L3_SW6_V1_20220211/CarMaker/VehicleControl/SDFADataLog/Subsystem94 ==
  BusCreator : BusCreator  Inputs=10
  Data Type Conversion{1..3,92} (4 alike) : DataTypeConversion  OutDataTypeStr=single
  Ground{,1..5} (6 alike) : Ground
  Read CM Dict1 : CarMaker4SL/Read CM Dict  xname=User.IO.Out.Orientation_S0_002  xsync=off
  Read CM Dict2 : CarMaker4SL/Read CM Dict  xname=User.IO.Out.Orientation_S0_003  xsync=off
  Read CM Dict3 : CarMaker4SL/Read CM Dict  xname=User.IO.Out.Orientation_S0_004  xsync=off
  Read CM Dict5 : CarMaker4SL/Read CM Dict  xname=User.IO.Out.Orientation_S0_001  xsync=off
  LBtar_Orientation : Outport
  wires:
  Data Type Conversion92/1 -> BusCreator/1
  Data Type Conversion1/1 -> BusCreator/2
  Data Type Conversion3/1 -> BusCreator/4
  Data Type Conversion2/1 -> BusCreator/3
  BusCreator/1 -> LBtar_Orientation/1
  Read CM Dict3/1 -> Data Type Conversion3/1
  Read CM Dict2/1 -> Data Type Conversion2/1
  Read CM Dict1/1 -> Data Type Conversion1/1
  Read CM Dict5/1 -> Data Type Conversion92/1
  Ground/1 -> BusCreator/5
  Ground1/1 -> BusCreator/6
  Ground2/1 -> BusCreator/7
  Ground3/1 -> BusCreator/8
  Ground4/1 -> BusCreator/9
  Ground5/1 -> BusCreator/10

== system MIL4L3_SW6_V1_20220211/CarMaker/VehicleControl/SDFADataLog/Subsystem95 ==
  BusCreator : BusCreator  Inputs=10
  Data Type Conversion{1..3,92} (4 alike) : DataTypeConversion  OutDataTypeStr=single
  Ground{,1..5} (6 alike) : Ground
  Read CM Dict1 : CarMaker4SL/Read CM Dict  xname=User.IO.Out.ExistenceProbability_S0_002  xsync=off
  Read CM Dict2 : CarMaker4SL/Read CM Dict  xname=User.IO.Out.ExistenceProbability_S0_003  xsync=off
  Read CM Dict3 : CarMaker4SL/Read CM Dict  xname=User.IO.Out.ExistenceProbability_S0_004  xsync=off
  Read CM Dict5 : CarMaker4SL/Read CM Dict  xname=User.IO.Out.ExistenceProbability_S0_001  xsync=off
  LBtar_ExistenceProbability : Outport
  wires:
  Data Type Conversion92/1 -> BusCreator/1
  Data Type Conversion2/1 -> BusCreator/3
  Data Type Conversion3/1 -> BusCreator/4
  Data Type Conversion1/1 -> BusCreator/2
  Ground5/1 -> BusCreator/10
  Ground4/1 -> BusCreator/9
  Ground3/1 -> BusCreator/8
  Ground2/1 -> BusCreator/7
  Ground1/1 -> BusCreator/6
  Ground/1 -> BusCreator/5
  Read CM Dict5/1 -> Data Type Conversion92/1
  Read CM Dict1/1 -> Data Type Conversion1/1
  Read CM Dict2/1 -> Data Type Conversion2/1
  Read CM Dict3/1 -> Data Type Conversion3/1
  BusCreator/1 -> LBtar_ExistenceProbability/1

== system MIL4L3_SW6_V1_20220211/CarMaker/VehicleControl/SDFADataLog/Subsystem96 ==
  BusCreator : BusCreator  Inputs=10
  Data Type Conversion{1..3,144} (4 alike) : DataTypeConversion  OutDataTypeStr=uint8
  Ground{,1..5} (6 alike) : Ground
  Read CM Dict1 : CarMaker4SL/Read CM Dict  xname=User.IO.Out.ClassHighest_S0_002  xsync=off
  Read CM Dict2 : CarMaker4SL/Read CM Dict  xname=User.IO.Out.ClassHighest_S0_003  xsync=off
  Read CM Dict3 : CarMaker4SL/Read CM Dict  xname=User.IO.Out.ClassHighest_S0_004  xsync=off
  Read CM Dict5 : CarMaker4SL/Read CM Dict  xname=User.IO.Out.ClassHighest_S0_001  xsync=off
  LBtar_Class : Outport
  wires:
  Data Type Conversion3/1 -> BusCreator/4
  Data Type Conversion2/1 -> BusCreator/3
  Data Type Conversion1/1 -> BusCreator/2
  Data Type Conversion144/1 -> BusCreator/1
  BusCreator/1 -> LBtar_Class/1
  Read CM Dict3/1 -> Data Type Conversion3/1
  Read CM Dict2/1 -> Data Type Conversion2/1
  Read CM Dict1/1 -> Data Type Conversion1/1
  Read CM Dict5/1 -> Data Type Conversion144/1
  Ground/1 -> BusCreator/5
  Ground1/1 -> BusCreator/6
  Ground2/1 -> BusCreator/7
  Ground3/1 -> BusCreator/8
  Ground4/1 -> BusCreator/9
  Ground5/1 -> BusCreator/10
